simulink model "Practica3"  (R2024b)
settings: Solver=VariableStepAuto  StartTime=0.0  StopTime=tsim  MaxStep=10/f  RelTol=1e-3
values from neighbouring files (symbols this model uses):
  f = 8e3    (= 8000)    [Practica_3.m]
  Kp = 0.001    [Practica_3.m]
  L1 = 0    [Practica_3.m]
  L2 = 0    [Practica_3.m]
  Lm = 0    [Practica_3.m]
  Pmp = 10524.2    [Practica_3.m]
  R1 = 0.1    [Practica_3.m]
  R2 = 0.1    [Practica_3.m]
  Rm = 10e6    (= 10000000)    [Practica_3.m]
  Ti = 30    [Practica_3.m]
  Tm = T/2    (= 6.25e-05)    [Practica_3.m]
  V1 = V2/2    (= 200)    [Practica_3.m]
  V2 = 400    [Practica_3.m]
  Vdc = 500    [Practica_3.m]
  Vmp = 223.836    [Practica_3.m]
libraries: spsCurrentMeasurementLib x4, spsVoltageMeasurementLib x3, spsParallelRLCBranchLib x2, spsDiodeLib x1, spsLinearTransformerLib x1, spsPVArrayLib x1, spsBistableLib x1, slpidlib x1, spsIGBTLib x1, simulink x1, spsDCVoltageSourceLib x1, sps_lib x1
settings Model: Creator=javier  LastModifiedBy=javier

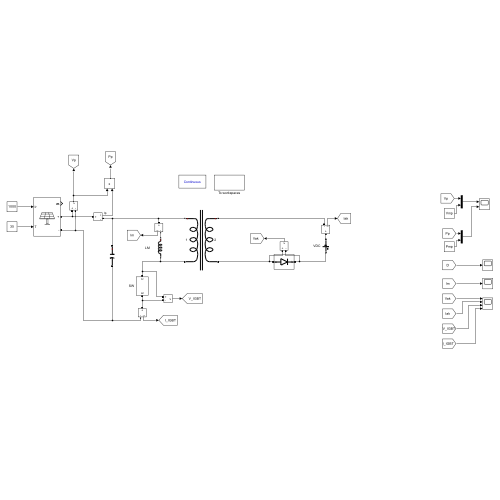
[thumbnail: Simulink's stored preview of the top-level diagram]
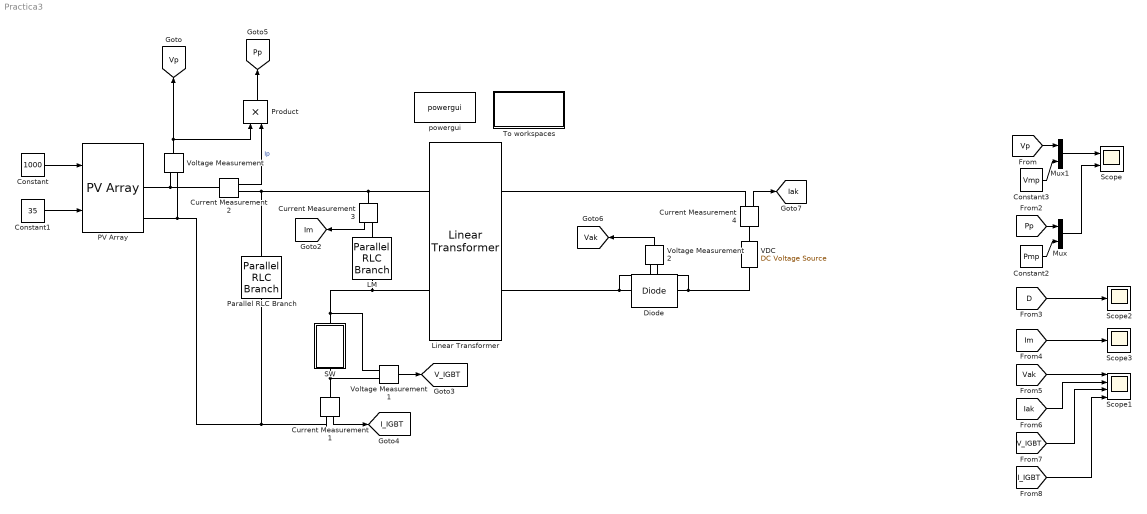
== system Practica3 ==
  Constant : Constant  Value=1000
  Constant1 : Constant  Value=35
  Constant2 : Constant  Value=Pmp
  Constant3 : Constant  Value=Vmp
  Current Measurement{1..4} (4 alike) : spsCurrentMeasurementLib/Current Measurement  PhasorSimulation=off  OutputType=Complex  PSBequivalent=0
  Diode : spsDiodeLib/Diode  Ron=0.001  Lon=0  Vf=0.8  IC=0  UseSnubber=0  Rs=500  Cs=250e-9  Measurements=off
  LM : spsParallelRLCBranchLib/Parallel RLC Branch  LConnTagsString=a  RConnTagsString=__new0  BranchType=L  Resistance=1  Inductance=2e-3  SetiL0=off  InitialCurrent=0  Capacitance=1.5e-3  Setx0=off  InitialVoltage=0  Measurements=None
  Linear Transformer : spsLinearTransformerLib/Linear Transformer  UNITS=SI  NominalPower=[Pmp f ]  winding1=[V1 R1 L1]  winding2=[V2 R2 L2]  ThreeWindings=off  winding3=[3.15e+05 0.7938 0.084225]  RmLm=[Rm Lm]  Measurements=None  DataType=on
  Mux : Mux  Inputs=2
  Mux1 : Mux  Inputs=2
  PV Array : spsPVArrayLib/PV Array  Npar=6  Nser=5  PlotType=array @ 1000 W/m2 & specified temperatures  S_vec=[1500]  Temp_C_vec=[35]  ModuleName=Solarbine SB-S370TA1  PlotWhenSelected=off  Pm=370.041  Ncell=96  Voc=58.28  Isc=8.36  Vm=46.9  Im=7.89  beta_Voc_pc=-0.37345  alpha_Isc_pc=0.010084  beta_Voc=-0.21765  alpha_Isc=0.000843  IL=8.3983  I0=4.1737e-10  nI=0.99638  Rsh=688.7261  Rs=0.53444  RobustModel=off  RobustCellTemperature=313.3991  BAL=on  Tc=1e-6  Tfilter=5e-5
  Parallel RLC Branch : spsParallelRLCBranchLib/Parallel RLC Branch  LConnTagsString=a  RConnTagsString=__new0  BranchType=C  Resistance=1  Inductance=1e-3  SetiL0=off  InitialCurrent=0  Capacitance=1.5e-3  Setx0=off  InitialVoltage=0  Measurements=None
  Product : Product
  SW : Subsystem
  Scope : Scope  NumInputPorts=2
  Scope1 : Scope  NumInputPorts=4
  Scope2 : Scope
  Scope3 : Scope
  To workspaces : Subsystem
  VDC : spsDCVoltageSourceLib/DC Voltage Source  Amplitude=Vdc  Measurements=None
  Voltage Measurement : spsVoltageMeasurementLib/Voltage Measurement  PhasorSimulation=off  OutputType=Complex  PSBequivalent=0
  Voltage Measurement1 : spsVoltageMeasurementLib/Voltage Measurement  PhasorSimulation=off  OutputType=Complex  PSBequivalent=0
  Voltage Measurement2 : spsVoltageMeasurementLib/Voltage Measurement  PhasorSimulation=off  OutputType=Complex  PSBequivalent=0
  powergui : sps_lib/powergui  Priority=1  SimulationMode=Continuous  SampleTime=50e-6  frequency=60  Iterations=50  frequencyindice=0  Pbase=100e6  ErrMax=1e-4  UnitsV=kV  UnitsW=MW  buscounter=0  FunctionMessages=off  echomessages=off  EnableUseOfTLC=off  CurrentSourceSwitches=off  DisableSnubberDevices=on  DisableRonSwitches=off  DisableVfSwitches=off  DisplayEquations=off  AutomaticDiscreteSolvers=off  SolverType=Tustin/Backward Euler (TBE)  Interpol=off  ExternalGateDelay=off  methode=off  Ts=100  x0status=blocks  SPID=on  SwTol=0  HookPort=off  NonlinearTolerance=1e-4  nMaxIteration=100  ContinueOnMaxIteration=off  RestoreLinks=warning  ResistiveCurrentMeasurement=off  Frange=[0:2:500]  Ylog=off  Xlog=on  ShowGrid=off  save=off  variable=ZData  structure=0  ZoomFFT=off  StartTime=0.0  cycles=1  DisplayStyle=1  fundamental=60  FreqAxis=off  MaxFrequency=1000  frequencyindicesteady=1  RmsSteady=1  display=off
  tag scope: I_IGBT=global, Iak=global, Im=global, Pp=global, V_IGBT=global, Vak=global, Vp=global
  wires:
  Constant1/1 -> PV Array/2
  Constant/1 -> PV Array/1
  Voltage Measurement/1 -> [Vp], Product/1
  Current Measurement1/1 -> [I_IGBT]
  Voltage Measurement1/1 -> [V_IGBT]
  Current Measurement2/1 -> Product/2  "Ip"
  Product/1 -> [Pp]
  Current Measurement3/1 -> [Im]
  Voltage Measurement2/1 -> [Vak]
  Current Measurement4/1 -> [Iak]
  [Im] -> Scope3/1
  Mux/1 -> Scope/2
  [Pp] -> Mux/1
  Constant2/1 -> Mux/2
  Mux1/1 -> Scope/1
  [Vp] -> Mux1/1
  Constant3/1 -> Mux1/2
  [D] -> Scope2/1
  [Vak] -> Scope1/1
  [Iak] -> Scope1/2
  [I_IGBT] -> Scope1/4
  [V_IGBT] -> Scope1/3
  connections:
  PV Array/RConn1 -- Current Measurement2/LConn1 -- Voltage Measurement/LConn1
  PV Array/RConn2 -- Voltage Measurement/LConn2 -- Current Measurement1/RConn1 -- Parallel RLC Branch/RConn1
  SW/LConn1 -- LM/RConn1 -- Linear Transformer/LConn2 -- Voltage Measurement1/LConn1
  Diode/LConn1 -- Linear Transformer/RConn2 -- Voltage Measurement2/LConn1
  Voltage Measurement2/LConn2 -- VDC/RConn1 -- Diode/RConn1
  Current Measurement1/LConn1 -- Voltage Measurement1/LConn2 -- SW/RConn1
  Linear Transformer/LConn1 -- Current Measurement3/LConn1 -- Parallel RLC Branch/LConn1 -- Current Measurement2/RConn1
  Current Measurement3/RConn1 -- LM/LConn1
  Current Measurement4/LConn1 -- VDC/LConn1
  Linear Transformer/RConn1 -- Current Measurement4/RConn1

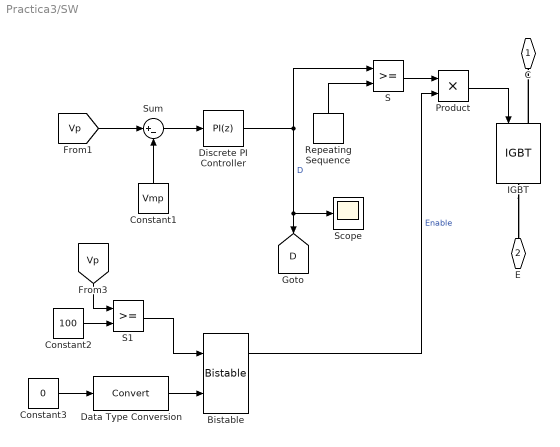
== system Practica3/SW ==
  Bistable : spsBistableLib/Bistable  Qpriority=Set  ic=0  Ts=0
      settings: LibrarySourceBlock=sps_lib/Control/Bistable
  Constant1 : Constant  Value=Vmp
  Constant2 : Constant  Value=100
  Constant3 : Constant  Value=0
  Data Type Conversion : DataTypeConversion  SaturateOnIntegerOverflow=off  RndMeth=Floor
  Discrete PI Controller : slpidlib/PID Controller  Controller=PI  Form=Ideal  TimeDomain=Discrete-time  UseExternalTs=off  SampleTime=Tm  IntegratorMethod=Forward Euler  FilterMethod=Forward Euler  ControllerParametersSource=internal  P=Kp  I=Ti  UseKiTs=off  D=0  UseExternalDerivativeSource=off  N=100  UseFilter=on  TunerSelectOption=Transfer Function Based (PID Tuner App)  InitialConditionSource=internal  InitialConditionForIntegrator=0  InitialConditionForFilter=0  DifferentiatorICPrevScaledInput=0  ExternalReset=none  TrackingMode=off  Kt=1  LimitOutput=off  SatLimitsSource=internal  UpperSaturationLimit=inf  LowerSaturationLimit=-inf  LinearizeAsGain=off  AntiWindupMode=none  Kb=1  LimitIntegrator=off  UpperIntegratorSaturationLimit=inf  LowerIntegratorSaturationLimit=-inf  POutMin=[]  POutMax=[]  IOutMin=[]  IOutMax=[]  DOutMin=[]  DOutMax=[]  NOutMin=[]  NOutMax=[]  SumOutMin=[]  SumOutMax=[]  SaturationOutMin=[]  SaturationOutMax=[]  PParamMin=[]  PParamMax=[]  IParamMin=[]  IParamMax=[]  DParamMin=[]  DParamMax=[]  NParamMin=[]  NParamMax=[]  KbParamMin=[]  KbParamMax=[]  KtParamMin=[]  KtParamMax=[]  KbOutMin=[]  KbOutMax=[]  KtOutMin=[]  KtOutMax=[]  IntegratorOutMin=[]  IntegratorOutMax=[]  FilterOutMin=[]  FilterOutMax=[]  SumI1OutMin=[]  SumI1OutMax=[]  SumI2OutMin=[]  SumI2OutMax=[]  SumI3OutMin=[]  SumI3OutMax=[]  SumI4OutMin=[]  SumI4OutMax=[]  SumDOutMin=[]  SumDOutMax=[]  DifferentiatorOutMin=[]  DifferentiatorOutMax=[]  FilterDiffOutCoefMin=[]  FilterDiffOutCoefMax=[]  ReciprocalOutMin=[]  ReciprocalOutMax=[]  SumDenOutMin=[]  SumDenOutMax=[]  SumNumOutMin=[]  SumNumOutMax=[]  DivideOutMin=[]  DivideOutMax=[]  UdiffTsProdOutMin=[]  UdiffTsProdOutMax=[]  NTsProdOutMin=[]  NTsProdOutMax=[]  UintegralTsProdOutMin=[]  UintegralTsProdOutMax=[]  UngainTsProdOutMin=[]  UngainTsProdOutMax=[]  ClampingZeroOutDataTypeStr=Inherit: Inherit via back propagation  ClampingZeroOutMin=[]  ClampingZeroOutMax=[]  FilterDenConstantOutDataTypeStr=Inherit: Inherit via back propagation  FilterDenConstantOutMin=[]  FilterDenConstantOutMax=[]  PCopyOutDataTypeStr=Inherit: Inherit via back propagation  PCopyOutMin=[]  PCopyOutMax=[]  NCopyOutDataTypeStr=Inherit: Inherit via back propagation  NCopyOutMin=[]  NCopyOutMax=[]  IntegratorContinuousStateAttributes=''  IntegratorStateMustResolveToSignalObject=off  IntegratorRTWStateStorageClass=Auto  FilterContinuousStateAttributes=''  FilterStateMustResolveToSignalObject=off  FilterRTWStateStorageClass=Auto  ParallelPVariant=Passthrough  IdealPVariant=InternalParameters  IVariant=InternalParameters  DVariant=Disabled  IntegratorVariant=Discrete  SatVariant=Disabled  AWVariant=Passthrough  PCopyVariant=Disabled  TRVariant=Disabled  FdbkBlocksVariant=Forward  IdealPFdbkVariant=Disabled  SatFdbkVariant=Disabled  DerivativeFilterVariant=Disabled  NVariant=Disabled  NCopyVariant=Disabled_SignalSpec  FilterICVariant=Disabled  IntegratorICVariant=InternalICs  ExternalResetVariant=Disabled  TRSumVariant=Passthrough  SumFdbkVariant=Disabled  SumVariant=Sum_PI  TsampFilterVariant=InternalTs  TsampNgainVariant=Passthrough  TsampIntegralVariant=Disabled_SignalSpec  ExternalSaturationOutDataTypeStr=Inherit: Same as second input  DerivativeSourceVariant=Disabled  PreIntVariant=InternalPreInt
  IGBT : spsIGBTLib/IGBT  Ron=0.001  Lon=0  Vf=1  Tf=1e-6  Tt=2e-6  IC=0  Rs=1e5  Cs=inf  Measurements=off
  Product : Product
  Repeating Sequence : simulink/Sources/Repeating Sequence  rep_seq_t=RepeatingTime  rep_seq_y=RepeatingOut
  S : RelationalOperator  OutDataTypeStr=boolean  RndMeth=Simplest  InputSameDT=off
  S1 : RelationalOperator  OutDataTypeStr=boolean  RndMeth=Simplest  InputSameDT=off
  Scope : Scope
  Sum : Sum  Inputs=|+-
  C : PMIOPort  Side=Left
  E : PMIOPort  Port=2  Side=Right
  tag scope: D=global
  wires:
  Discrete PI Controller/1 -> Scope/1, [D], S/1  "D"
  Repeating Sequence/1 -> S/2
  Sum/1 -> Discrete PI Controller/1
  [Vp] -> Sum/1
  Constant1/1 -> Sum/2
  Product/1 -> IGBT/1
  S/1 -> Product/1
  Bistable/1 -> Product/2  "Enable"
  Constant3/1 -> Data Type Conversion/1
  [Vp] -> S1/1
  Data Type Conversion/1 -> Bistable/2
  S1/1 -> Bistable/1
  Constant2/1 -> S1/2
  connections:
  IGBT/RConn1 -- E/RConn1
  IGBT/LConn1 -- C/RConn1

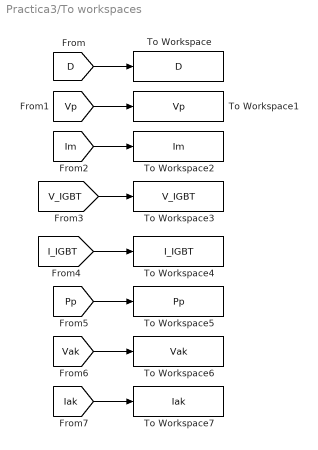
== system Practica3/To workspaces ==
  To Workspace : ToWorkspace  VariableName=D  SaveFormat=Timeseries  SampleTime=-1
  To Workspace1 : ToWorkspace  VariableName=Vp  SaveFormat=Timeseries  SampleTime=-1
  To Workspace2 : ToWorkspace  VariableName=Im  SaveFormat=Timeseries  SampleTime=-1
  To Workspace3 : ToWorkspace  VariableName=V_IGBT  SaveFormat=Timeseries  SampleTime=-1
  To Workspace4 : ToWorkspace  VariableName=I_IGBT  SaveFormat=Timeseries  SampleTime=-1
  To Workspace5 : ToWorkspace  VariableName=Pp  SaveFormat=Timeseries  SampleTime=-1
  To Workspace6 : ToWorkspace  VariableName=Vak  SaveFormat=Timeseries  SampleTime=-1
  To Workspace7 : ToWorkspace  VariableName=Iak  SaveFormat=Timeseries  SampleTime=-1
  wires:
  [V_IGBT] -> To Workspace3/1
  [Im] -> To Workspace2/1
  [Pp] -> To Workspace5/1
  [I_IGBT] -> To Workspace4/1
  [Vp] -> To Workspace1/1
  [D] -> To Workspace/1
  [Vak] -> To Workspace6/1
  [Iak] -> To Workspace7/1
